simulink model "NonLinNomoto2"  (R2015b)
settings: Solver=VariableStepAuto  StartTime=0.0  StopTime=tstop  FixedStep=0.01  RelTol=1e-3
values from neighbouring files (symbols this model uses):
  b_1 = [800009.963225 12.8568262477]    [H_b_curvefitting.mat]    (also in Yaw and Yaw-rate controller.mat = [800009.882282 13.5298731691]; Yaw_NonLin_controller.mat; analyse_ulin_dynamics kopi.m = lsqcurvefit(F5, b_1_0, r_list_c, d_list,[],[],OPT); analyse_ulin_dynamics.m = lsqcurvefit(F5, b_1_0, r_list_c, d_list,[1e5 0],[inf inf],OP)
  b_2 = [1209648.76119 1.27157024962e-10 288.459050574]    [H_b_curvefitting.mat]    (also in Yaw and Yaw-rate controller.mat = [1233422.7042 3.06871796591e-14 291.893339409]; Yaw_NonLin_controller.mat = [1209648.75063 1.2654213265e-10 288.459058131]; analyse_ulin_dynamics kopi.m = lsqcurvefit(F6, b_2_0, r_list_c, d_list,[0 0 0],[],OPT); analyse_ulin_dynamics.m = lsqcurvefit(F6, b_2_0, r_list_c, d_list,[1e5 0 0],[inf inf i)
  delta_c = dc_list(i)    [NonLinearAnalysis.m]    (also in Run_Delta_R_Sim.m = d_list(i); analyse_lin_dynamics.m = deg2rad(delta_list(i)); analyse_ulin_dynamics kopi.m = deg2rad(delta); analyse_ulin_dynamics.m = deg2rad(delta_list(i)))
  tsamp = 10    [NonLinearAnalysis.m]    (also in analyse_lin_dynamics.m = 20; analyse_steadystate.m; analyse_ulin_dynamics kopi.m; analyse_ulin_dynamics.m)
  x = lsqcurvefit(F4, x0, t, r,[20 0],[500 0.15],OPT)    [analyse_lin_dynamics.m]    (also in analyse_ulin_dynamics kopi.m = lsqcurvefit(F8, x0, t, r,[],[],OPT); analyse_ulin_dynamics.m = lsqcurvefit(F8, x0, t, r,[0 0],[400 1],OPT); curvefitting.m = lsqcurvefit(F, x0, t, r); run.m = lsqcurvefit(F_4, x0, t, r))
undefined symbols (not defined in the file or in its folder): b_3
settings Model: Creator=Erik  LastModifiedBy=Erik
settings HardwareCC: ProdBitPerPointer=32  ProdLargestAtomicFloat=None  ProdIntDivRoundTo=Undefined  ProdEndianess=Unspecified  ProdWordSize=32  ProdHWDeviceType=32-bit Generic
settings GRTTargetCC: GeneratePreprocessorConditionals=Disable all

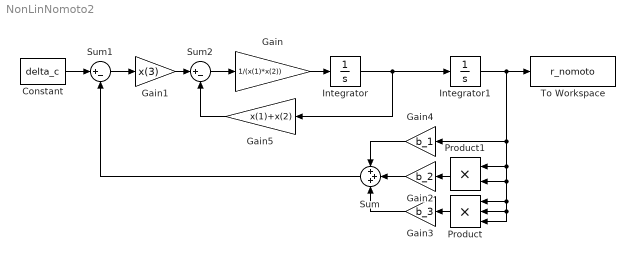
== system NonLinNomoto2 ==
  Constant : Constant  Value=delta_c
  Gain : Gain  Gain=1/(x(1)*x(2))
  Gain1 : Gain  Gain=x(3)
  Gain2 : Gain  Gain=b_2
  Gain3 : Gain  Gain=b_3
  Gain4 : Gain  Gain=b_1
  Gain5 : Gain  Gain=x(1)+x(2)
  Integrator : Integrator
  Integrator1 : Integrator
  Product : Product  Inputs=3
  Product1 : Product
  Sum : Sum  Inputs=+++
  Sum1 : Sum  Inputs=|+-
  Sum2 : Sum  Inputs=|+-
  To Workspace : ToWorkspace  VariableName=r_nomoto  SampleTime=tsamp
  wires:
  Integrator/1 -> Gain5/1, Integrator1/1
  Product/1 -> Gain3/1
  Integrator1/1 -> To Workspace/1, Product1/1, Product1/2, Product/3, Product/2, Product/1, Gain4/1
  Gain/1 -> Integrator/1
  Constant/1 -> Sum1/1
  Sum1/1 -> Gain1/1
  Gain4/1 -> Sum/1
  Sum/1 -> Sum1/2
  Gain1/1 -> Sum2/1
  Sum2/1 -> Gain/1
  Gain5/1 -> Sum2/2
  Product1/1 -> Gain2/1
  Gain3/1 -> Sum/3
  Gain2/1 -> Sum/2
